simulink subsystem "roll_controller"  (R2024b)
settings: Solver=VariableStepAuto  StartTime=0.0  StopTime=10.0  RelTol=1e-3
settings Model: Creator=yagiz  LastModifiedBy=yagiz

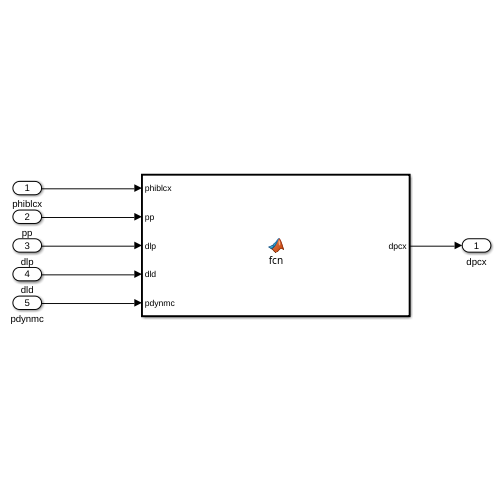
[thumbnail: Simulink's stored preview of the top-level diagram]
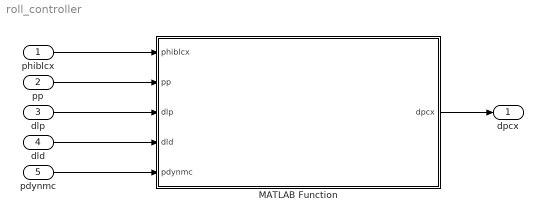
== system roll_controller ==
  phiblcx : Inport
  pp : Inport  Port=2
  dlp : Inport  Port=3
  dld : Inport  Port=4
  pdynmc : Inport  Port=5
  MATLAB Function : MATLAB Function  TreatAsAtomicUnit=on
  dpcx : Outport
  wires:
  phiblcx/1 -> MATLAB Function/1(phiblcx)
  pp/1 -> MATLAB Function/2(pp)
  dlp/1 -> MATLAB Function/3(dlp)
  dld/1 -> MATLAB Function/4(dld)
  pdynmc/1 -> MATLAB Function/5(pdynmc)
  MATLAB Function/1(dpcx) -> dpcx/1

== matlab function roll_controller/MATLAB Function ==
  data: phiblcx input; dpcx output; pp input; dlp input; dld input; pdynmc input
function dpcx  = fcn(phiblcx, pp, dlp, dld, pdynmc)

zrcl     = 0.9;
factwrcl = 0.0;
phicomx  = 0.0;   % commanded roll = 0 (level flight)
DEG = 180/pi;

% Variable roll bandwidth
wrcl = (0.00024 * pdynmc + 10.0) * (1.0 + factwrcl);

% Gains
gkp   = (2.0 * zrcl * wrcl + dlp) / dld;
gkphi = wrcl * wrcl / dld;

% Roll position command
ephi = gkphi * (phicomx - phiblcx) * (pi/180);
dpc  = ephi - gkp * pp;
dpcx = dpc * DEG;

% Limit
dplimx = 28.0;
dpcx = max(-dplimx, min(dplimx, dpcx));
